simulink model "SITL"  (R2015a)
settings: Solver=ode3  StartTime=0.0  StopTime=tempofinal  FixedStep=0.02  RelTol=1e-3
values from neighbouring files (symbols this model uses):
  controle = 0    [main_quad.m]
  cq = 2.4086*10^(-7)    (= 2.4086e-07)    [main_quad.m]
  ct = 1.4341*10^(-5)    (= 1.4341e-05)    [main_quad.m]
  d = 0.26    [main_quad.m]
  g = 9.8065    [main_quad.m]
  J = [Jxx,Jyy,Jzz,Jm]    [main_quad.m]
  Ja = 5e-5    (= 5e-05)    [main_quad.m]
  k1 = 2.5    [main_quad.m]
  k2 = 6.2360    (= 6.236)    [main_quad.m]
  k3 = 6.2360    (= 6.236)    [main_quad.m]
  k4 = 0.4927    [main_quad.m]
  k5 = 1.6    [main_quad.m]
  k6 = 1.6    [main_quad.m]
  ke = kt    (= 0.024)    [main_quad.m]
  kt = 0.024    [main_quad.m]
  lambda1 = 1    [main_quad.m]
  lambda2 = 5    [main_quad.m]
  lambda3 = 5    [main_quad.m]
  lambda4 = 1/2    (= 0.5)    [main_quad.m]
  lambda5 = 1/4    (= 0.25)    [main_quad.m]
  lambda6 = 1/4    (= 0.25)    [main_quad.m]
  limit = [0.5 0.5 0.5 0.5]    [main_quad.m]
  limit_pos = [0.5 0.5]    [main_quad.m]
  m = 1.03    [main_quad.m]
  max_w = 733.03    [main_quad.m]
  Pitch_D = 0.019    [main_quad.m]
  Pitch_P = 0.019948    [main_quad.m]
  pos_D = -0.033991    [main_quad.m]
  pos_P = -0.005948    [main_quad.m]
  R = 0.2    [main_quad.m]    (also in plot_resultados.m = A(:,12))
  Roll_D = 0.019    [main_quad.m]
  Roll_P = 0.019948    [main_quad.m]
  w1_0 = w_hover    [main_quad.m]
  w2_0 = w_hover    [main_quad.m]
  w3_0 = w_hover    [main_quad.m]
  w4_0 = w_hover    [main_quad.m]
  X = A(:,1)    [plot_resultados.m]
  Yaw_D = 0.037200    (= 0.0372)    [main_quad.m]
  Yaw_P = 0.039055    [main_quad.m]
  Z_D = -0.682000    (= -0.682)    [main_quad.m]
  Z_P = -0.238672    [main_quad.m]
undefined symbols (not defined in the file or in its folder): selecting_parameters
libraries: dspnetwork x2, etargetslib x2
settings Model: Creator=Adriano  LastModifiedBy=Andre
settings DebuggingCC: UnderspecifiedInitializationDetection=Classic  MergeDetectMultiDrivingBlocksExec=none  SolverPrmCheckMsg=warning  StateNameClashWarn=warning
settings HardwareCC: ProdLargestAtomicInteger=Long  ProdLargestAtomicFloat=Double  ProdIntDivRoundTo=Floor  ProdEndianess=LittleEndian  ProdHWDeviceType=ARM Compatible->ARM Cortex
settings RTWCC: GenerateReport=on  LaunchReport=on
settings GRTTargetCC: CodeReplacementLibrary=GNU C99 extensions  RTWCAPISignals=on  RTWCAPIParams=on

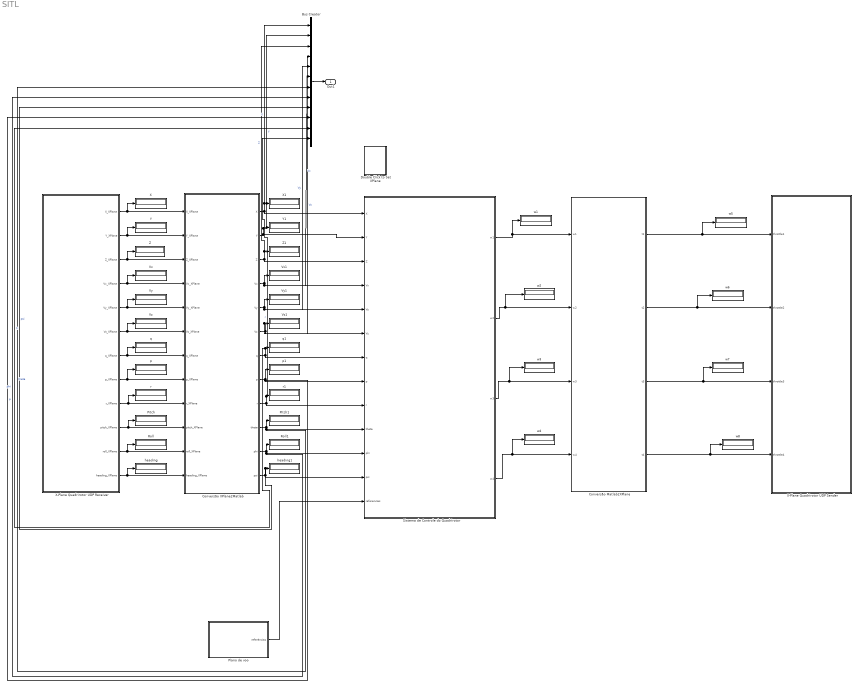
== system SITL ==
  Bus Creator : BusCreator  Inputs=12
  Conversão Matlab2XPlane : Subsystem
  Conversão XPlane2Matlab : Subsystem
  Double Click to Set XPlane : Subsystem  LoadFcn=selecting_parameters()
      settings: OpenFcn=selecting_parameters()
  Pitch : Display
  Pitch1 : Display
  Plano de voo : Subsystem
  Roll : Display
  Roll1 : Display
  Sistema de Controle do Quadrirotor : Subsystem
  Vx : Display
  Vx1 : Display
  Vy : Display
  Vy1 : Display
  Vz : Display
  Vz1 : Display
  X : Display
  X-Plane Quadrirotor UDP Receiver : Subsystem  AncestorBlock=X_Plane_Communication_Library/Fixed Wing/X-Plane Fixed Wing UDP Receiver  mask{ip_adress='127.0.0.1', port_number=49004}
      mask prompts: ip_adress "Local IP Adress (default: '127.0.0.1' )"; port_number "Output Port Number (defaut: '49004')"
      mask help: This block is configured to receiver data from a fixed wing aircraft on X-Plane Flight Simulator.
      mask Help: Contact adrianobittar@gmail.com
  X-Plane Quadrirotor UDP Sender : Subsystem  AncestorBlock=X_Plane_Communication_Library/Fixed Wing/X-Plane Fixed Wing UDP Sender  mask{ip_adress='127.0.0.1', port_number=49000}
      mask prompts: ip_adress "Local IP Adress (default: '127.0.0.1' )"; port_number "Output Port Number (defaut: '49000')"
      mask help: This block is configured to send data to a fixed wing aircraft on X-Plane Flight Simulator.
      mask Help: Contact adrianobittar@gmail.com
  X1 : Display
  Y : Display
  Y1 : Display
  Z : Display
  Z1 : Display
  heading : Display
  heading1 : Display
  p : Display
  p1 : Display
  q : Display
  q1 : Display
  r : Display
  r1 : Display
  w{1..8} (8 alike) : Display
  Out1 : Outport
  wires:
  X-Plane Quadrirotor UDP Receiver/10(pitch_XPlane) -> Pitch/1, Conversão XPlane2Matlab/10(pitch_XPlane)
  X-Plane Quadrirotor UDP Receiver/1("X_XPlane ") -> X/1, Conversão XPlane2Matlab/1(X_XPlane)
  X-Plane Quadrirotor UDP Receiver/2(Y_XPlane) -> Conversão XPlane2Matlab/2(Y_XPlane), Y/1
  X-Plane Quadrirotor UDP Receiver/3(Z_XPlane) -> Conversão XPlane2Matlab/3(Z_XPlane), Z/1
  X-Plane Quadrirotor UDP Receiver/4(Vx_XPlane) -> Conversão XPlane2Matlab/4(Vx_XPlane), Vx/1
  X-Plane Quadrirotor UDP Receiver/5(Vy_XPlane) -> Conversão XPlane2Matlab/5(Vy_XPlane), Vy/1
  X-Plane Quadrirotor UDP Receiver/8(p_XPlane) -> Conversão XPlane2Matlab/8(p_XPlane), p/1
  X-Plane Quadrirotor UDP Receiver/11(roll_XPlane) -> Conversão XPlane2Matlab/11(roll_XPlane), Roll/1
  X-Plane Quadrirotor UDP Receiver/9(r_XPlane) -> Conversão XPlane2Matlab/9(r_XPlane), r/1
  X-Plane Quadrirotor UDP Receiver/6(Vz_XPlane) -> Conversão XPlane2Matlab/6(Vz_XPlane), Vz/1
  X-Plane Quadrirotor UDP Receiver/12(heading_XPlane) -> Conversão XPlane2Matlab/12(heading_XPlane), heading/1
  X-Plane Quadrirotor UDP Receiver/7(q_XPlane) -> Conversão XPlane2Matlab/7(q_XPlane), q/1
  Sistema de Controle do Quadrirotor/3(w3) -> Conversão Matlab2XPlane/3(w3), w3/1
  Sistema de Controle do Quadrirotor/4(w4) -> Conversão Matlab2XPlane/4(w4), w4/1
  Sistema de Controle do Quadrirotor/2(w2) -> Conversão Matlab2XPlane/2(w2), w2/1
  Sistema de Controle do Quadrirotor/1(w1) -> Conversão Matlab2XPlane/1(w1), w1/1
  Conversão XPlane2Matlab/12(psi) -> Bus Creator/9, heading1/1, Sistema de Controle do Quadrirotor/12(psi)  "psi"
  Conversão XPlane2Matlab/11(phi) -> Bus Creator/8, Sistema de Controle do Quadrirotor/11(phi), Roll1/1  "phi"
  Conversão XPlane2Matlab/10(theta) -> Bus Creator/7, Sistema de Controle do Quadrirotor/10(theta), Pitch1/1  "theta"
  Conversão XPlane2Matlab/9(r) -> Bus Creator/12, r1/1, Sistema de Controle do Quadrirotor/9(r)  "r"
  Conversão XPlane2Matlab/8(p) -> Sistema de Controle do Quadrirotor/8(p), Bus Creator/10, p1/1  "p"
  Conversão XPlane2Matlab/7(q) -> Bus Creator/11, q1/1, Sistema de Controle do Quadrirotor/7(q)  "q"
  Conversão XPlane2Matlab/6(Vz) -> Bus Creator/6, Vz1/1, Sistema de Controle do Quadrirotor/6(Vz)  "Vz"
  Conversão XPlane2Matlab/5(Vy) -> Sistema de Controle do Quadrirotor/5(Vy), Bus Creator/5, Vy1/1  "Vy"
  Conversão XPlane2Matlab/4(Vx) -> Sistema de Controle do Quadrirotor/4(Vx), Bus Creator/4, Vx1/1  "Vx"
  Conversão XPlane2Matlab/3(Z) -> Bus Creator/3, Z1/1, Sistema de Controle do Quadrirotor/3(Z)  "Z"
  Conversão XPlane2Matlab/2(Y) -> Bus Creator/2, Y1/1, Sistema de Controle do Quadrirotor/2(Y)  "Y"
  Conversão XPlane2Matlab/1("X ") -> Bus Creator/1, X1/1, Sistema de Controle do Quadrirotor/1(X)  "X"
  Conversão Matlab2XPlane/1(t1) -> w5/1, X-Plane Quadrirotor UDP Sender/1(throttle1)
  Conversão Matlab2XPlane/2(t2) -> w6/1, X-Plane Quadrirotor UDP Sender/2(throttle2)
  Conversão Matlab2XPlane/3(t3) -> w7/1, X-Plane Quadrirotor UDP Sender/3(throttle3)
  Conversão Matlab2XPlane/4(t4) -> w8/1, X-Plane Quadrirotor UDP Sender/4(throttle4)
  Plano de voo/1("referências ") -> Sistema de Controle do Quadrirotor/13(referencias)
  Bus Creator/1 -> Out1/1

== system SITL/Conversão Matlab2XPlane ==
  w1 : Inport
  w2 : Inport  Port=2
  w3 : Inport  Port=3
  w4 : Inport  Port=4
  MATLAB Function : MATLAB Function  TreatAsAtomicUnit=on
  t1 : Outport
  t2 : Outport  Port=2
  t3 : Outport  Port=3
  t4 : Outport  Port=4
  wires:
  w1/1 -> MATLAB Function/1(w1)
  w2/1 -> MATLAB Function/2(w2)
  w3/1 -> MATLAB Function/3(w3)
  w4/1 -> MATLAB Function/4(w4)
  MATLAB Function/1(t1) -> t1/1
  MATLAB Function/2(t2) -> t2/1
  MATLAB Function/3(t3) -> t3/1
  MATLAB Function/4(t4) -> t4/1

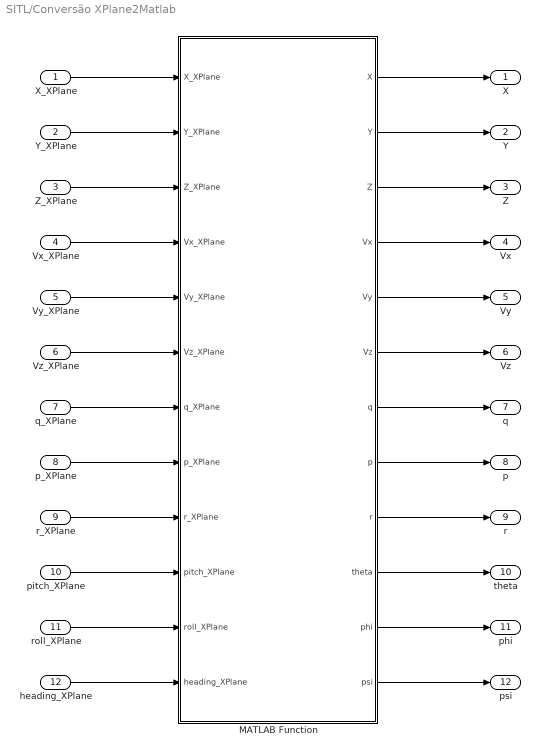
== system SITL/Conversão XPlane2Matlab ==
  X_XPlane : Inport
  Y_XPlane : Inport  Port=2
  Z_XPlane : Inport  Port=3
  Vx_XPlane : Inport  Port=4
  Vy_XPlane : Inport  Port=5
  Vz_XPlane : Inport  Port=6
  q_XPlane : Inport  Port=7
  p_XPlane : Inport  Port=8
  r_XPlane : Inport  Port=9
  pitch_XPlane : Inport  Port=10
  roll_XPlane : Inport  Port=11
  heading_XPlane : Inport  Port=12
  MATLAB Function : MATLAB Function  TreatAsAtomicUnit=on
  "X " : Outport
  Y : Outport  Port=2
  Z : Outport  Port=3
  Vx : Outport  Port=4
  Vy : Outport  Port=5
  Vz : Outport  Port=6
  q : Outport  Port=7
  p : Outport  Port=8
  r : Outport  Port=9
  theta : Outport  Port=10
  phi : Outport  Port=11
  psi : Outport  Port=12
  wires:
  MATLAB Function/12(psi) -> psi/1
  MATLAB Function/11(phi) -> phi/1
  MATLAB Function/10(theta) -> theta/1
  MATLAB Function/9(r) -> r/1
  MATLAB Function/8(p) -> p/1
  MATLAB Function/7(q) -> q/1
  MATLAB Function/6(Vz) -> Vz/1
  MATLAB Function/5(Vy) -> Vy/1
  MATLAB Function/4(Vx) -> Vx/1
  MATLAB Function/3(Z) -> Z/1
  MATLAB Function/2(Y) -> Y/1
  MATLAB Function/1(X) -> "X "/1
  X_XPlane/1 -> MATLAB Function/1(X_XPlane)
  Y_XPlane/1 -> MATLAB Function/2(Y_XPlane)
  Z_XPlane/1 -> MATLAB Function/3(Z_XPlane)
  Vx_XPlane/1 -> MATLAB Function/4(Vx_XPlane)
  Vy_XPlane/1 -> MATLAB Function/5(Vy_XPlane)
  Vz_XPlane/1 -> MATLAB Function/6(Vz_XPlane)
  q_XPlane/1 -> MATLAB Function/7(q_XPlane)
  p_XPlane/1 -> MATLAB Function/8(p_XPlane)
  r_XPlane/1 -> MATLAB Function/9(r_XPlane)
  pitch_XPlane/1 -> MATLAB Function/10(pitch_XPlane)
  roll_XPlane/1 -> MATLAB Function/11(roll_XPlane)
  heading_XPlane/1 -> MATLAB Function/12(heading_XPlane)

== system SITL/Double Click to Set XPlane ==

== system SITL/Plano de voo ==
  Gain1 : Gain
  Gain2 : Gain
  Gain3 : Gain  Gain=-1
  Gain4 : Gain
  Mux : Mux
  Step1 : Step  Time=30  After=150*pi/180  SampleTime=0
  Step2 : Step  Time=0  After=6  SampleTime=0
  Step_x : Step  Time=20  After=15  SampleTime=0
  Step_y : Step  Time=10  After=15  SampleTime=0
  "referências " : Outport
  wires:
  Mux/1 -> "referências "/1
  Gain3/1 -> Mux/3  "ref_z"
  Gain2/1 -> Mux/2  "ref_y"
  Gain4/1 -> Mux/1  "ref_x"
  Gain1/1 -> Mux/4  "ref_psi"
  Step1/1 -> Gain1/1
  Step2/1 -> Gain3/1
  Step_y/1 -> Gain2/1
  Step_x/1 -> Gain4/1

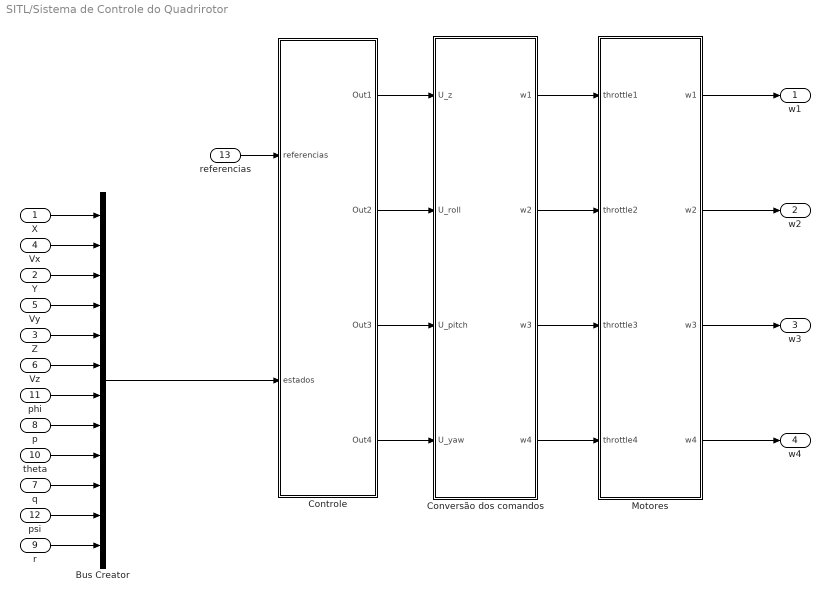
== system SITL/Sistema de Controle do Quadrirotor ==
  X : Inport
  Y : Inport  Port=2
  Z : Inport  Port=3
  Vx : Inport  Port=4
  Vy : Inport  Port=5
  Vz : Inport  Port=6
  q : Inport  Port=7
  p : Inport  Port=8
  r : Inport  Port=9
  theta : Inport  Port=10
  phi : Inport  Port=11
  psi : Inport  Port=12
  referencias : Inport  Port=13
  Bus Creator : BusCreator  Inputs=12
  Controle : Subsystem
  Conversão dos comandos : Subsystem
  Motores : Subsystem
  w1 : Outport
  w2 : Outport  Port=2
  w3 : Outport  Port=3
  w4 : Outport  Port=4
  wires:
  Conversão dos comandos/1(w1) -> Motores/1(throttle1)
  Conversão dos comandos/2(w2) -> Motores/2(throttle2)
  Conversão dos comandos/3(w3) -> Motores/3(throttle3)
  Conversão dos comandos/4(w4) -> Motores/4(throttle4)
  Controle/1(Out1) -> Conversão dos comandos/1(U_z)
  Controle/2(Out2) -> Conversão dos comandos/2(U_roll)
  Controle/3(Out3) -> Conversão dos comandos/3(U_pitch)
  Controle/4(Out4) -> Conversão dos comandos/4(U_yaw)
  referencias/1 -> Controle/1(referencias)
  X/1 -> Bus Creator/1
  Bus Creator/1 -> Controle/2(estados)
  Vx/1 -> Bus Creator/2
  Y/1 -> Bus Creator/3
  Vy/1 -> Bus Creator/4
  Z/1 -> Bus Creator/5
  Vz/1 -> Bus Creator/6
  phi/1 -> Bus Creator/7
  p/1 -> Bus Creator/8
  theta/1 -> Bus Creator/9
  q/1 -> Bus Creator/10
  psi/1 -> Bus Creator/11
  r/1 -> Bus Creator/12
  Motores/1(w1) -> w1/1
  Motores/2(w2) -> w2/1
  Motores/3(w3) -> w3/1
  Motores/4(w4) -> w4/1

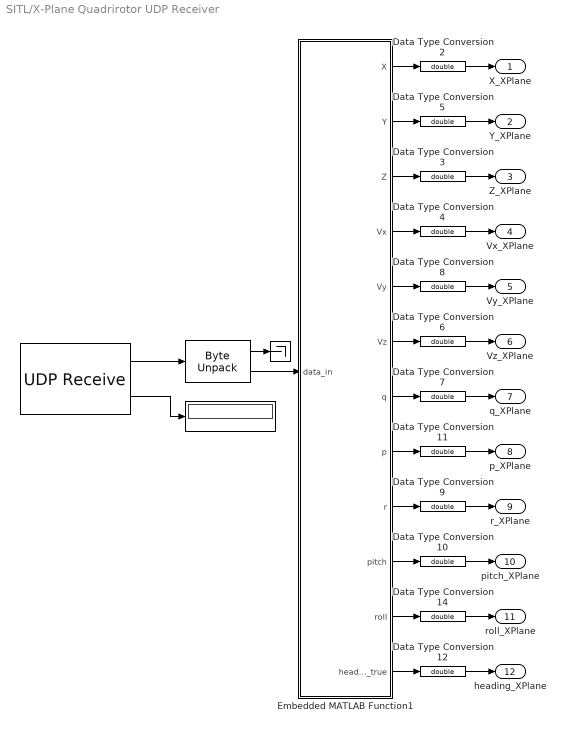
== system SITL/X-Plane Quadrirotor UDP Receiver ==
  " " : Display
  " " : Terminator
  "    " : dspnetwork/UDP Receive  localURL='0.0.0.0'  localPort=port_number  remoteURL=ip_adress  remotePort=-1  recvBufferSize=8192  dims=113  signalDatatype=uint8  isVarSize=off  showBlockingTime=on  blockingTime=1  sampletime=0.02  blockPlatform=WINDOWS
  "     " : etargetslib/Byte Unpack  dimensions={5,[9,3]}  datatypes={'uint8','single'}  byteAlign=1
  Data Type Conversion{2..12,14} (12 alike) : DataTypeConversion  OutDataTypeStr=double  SaturateOnIntegerOverflow=on
  Embedded MATLAB Function1 : MATLAB Function  TreatAsAtomicUnit=on
  "X_XPlane " : Outport
  Y_XPlane : Outport  Port=2
  Z_XPlane : Outport  Port=3
  Vx_XPlane : Outport  Port=4
  Vy_XPlane : Outport  Port=5
  Vz_XPlane : Outport  Port=6
  q_XPlane : Outport  Port=7
  p_XPlane : Outport  Port=8
  r_XPlane : Outport  Port=9
  pitch_XPlane : Outport  Port=10
  roll_XPlane : Outport  Port=11
  heading_XPlane : Outport  Port=12
  wires:
  Data Type Conversion11/1 -> p_XPlane/1
  Data Type Conversion14/1 -> roll_XPlane/1
  Data Type Conversion12/1 -> heading_XPlane/1
  Data Type Conversion7/1 -> q_XPlane/1
  Data Type Conversion6/1 -> Vz_XPlane/1
  Data Type Conversion4/1 -> Vx_XPlane/1
  Data Type Conversion3/1 -> Z_XPlane/1
  Data Type Conversion8/1 -> Vy_XPlane/1
  Data Type Conversion5/1 -> Y_XPlane/1
  Data Type Conversion2/1 -> "X_XPlane "/1
  Embedded MATLAB Function1/1(X) -> Data Type Conversion2/1
  Embedded MATLAB Function1/2(Y) -> Data Type Conversion5/1
  Embedded MATLAB Function1/3(Z) -> Data Type Conversion3/1
  Embedded MATLAB Function1/4(Vx) -> Data Type Conversion4/1
  Embedded MATLAB Function1/5(Vy) -> Data Type Conversion8/1
  Embedded MATLAB Function1/6(Vz) -> Data Type Conversion6/1
  Embedded MATLAB Function1/7(q) -> Data Type Conversion7/1
  Embedded MATLAB Function1/8(p) -> Data Type Conversion11/1
  Embedded MATLAB Function1/9(r) -> Data Type Conversion9/1
  Embedded MATLAB Function1/10(pitch) -> Data Type Conversion10/1
  Embedded MATLAB Function1/11(roll) -> Data Type Conversion14/1
  Embedded MATLAB Function1/12(heading_true) -> Data Type Conversion12/1
  "     "/1 -> " "/1
  "    "/2 -> " "/1
  Data Type Conversion10/1 -> pitch_XPlane/1
  "    "/1 -> "     "/1
  Data Type Conversion9/1 -> r_XPlane/1
  "     "/2 -> Embedded MATLAB Function1/1(data_in)

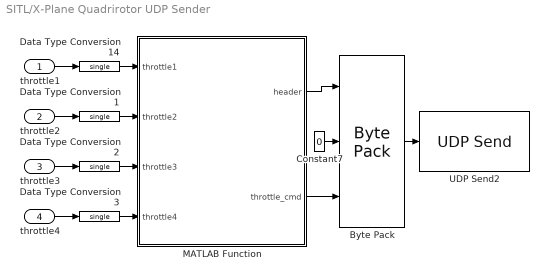
== system SITL/X-Plane Quadrirotor UDP Sender ==
  throttle1 : Inport
  throttle2 : Inport  Port=2
  throttle3 : Inport  Port=3
  throttle4 : Inport  Port=4
  Byte Pack : etargetslib/Byte Pack  datatypes={'single','uint8','single'}  byteAlign=1
  Constant7 : Constant  Value=0  OutDataTypeStr=uint8
  Data Type Conversion{1..3,14} (4 alike) : DataTypeConversion  OutDataTypeStr=single  SaturateOnIntegerOverflow=on
  MATLAB Function : MATLAB Function  TreatAsAtomicUnit=on
  UDP Send2 : dspnetwork/UDP Send  remoteURL=ip_adress  remotePort=port_number  localURL='255.255.255.255'  localPortSource=Automatically determine  localPort=-1  sampletime=-1  blockPlatform=HOST  separateLengthPort=0
  wires:
  Byte Pack/1 -> UDP Send2/1
  MATLAB Function/1(header) -> Byte Pack/1
  Data Type Conversion14/1 -> MATLAB Function/1(throttle1)
  throttle1/1 -> Data Type Conversion14/1
  Constant7/1 -> Byte Pack/2
  Data Type Conversion1/1 -> MATLAB Function/2(throttle2)
  Data Type Conversion2/1 -> MATLAB Function/3(throttle3)
  Data Type Conversion3/1 -> MATLAB Function/4(throttle4)
  throttle2/1 -> Data Type Conversion1/1
  throttle3/1 -> Data Type Conversion2/1
  throttle4/1 -> Data Type Conversion3/1
  MATLAB Function/2(throttle_cmd) -> Byte Pack/3

== system SITL/Sistema de Controle do Quadrirotor/Controle ==
  note: 0: controle Sliding Mode
      | 1: controle PD
  referencias : Inport
  estados : Inport  Port=2
  Constant : Constant  Value=0
  Controlador PD : Subsystem
  Controlador sliding mode : Subsystem
  Demux : Demux
  Switch : Switch  Criteria=u2 > Threshold
  Out1 : Outport
  Out2 : Outport  Port=2
  Out3 : Outport  Port=3
  Out4 : Outport  Port=4
  wires:
  referencias/1 -> Controlador sliding mode/1(Referências), Controlador PD/1(Referências)
  estados/1 -> Controlador sliding mode/2(Estados), Controlador PD/2(Estados)
  Switch/1 -> Demux/1
  Demux/1 -> Out1/1  "U_T"
  Demux/2 -> Out2/1  "U_L"
  Constant/1 -> Switch/2
  Demux/3 -> Out3/1  "U_M"
  Demux/4 -> Out4/1  "U_N"
  Controlador PD/1(Out1) -> Switch/1
  Controlador sliding mode/1(Out1) -> Switch/3

== system SITL/Sistema de Controle do Quadrirotor/Conversão dos comandos ==
  U_z : Inport
  U_roll : Inport  Port=2
  U_pitch : Inport  Port=3
  U_yaw : Inport  Port=4
  Constant1 : Constant  Value=ct
  Constant2 : Constant  Value=cq
  Constant4 : Constant  Value=d
  MATLAB Function : MATLAB Function  TreatAsAtomicUnit=on
  w1 : Outport
  w2 : Outport  Port=2
  w3 : Outport  Port=3
  w4 : Outport  Port=4
  wires:
  U_pitch/1 -> MATLAB Function/3(u_M)
  U_z/1 -> MATLAB Function/1(u_T)
  U_yaw/1 -> MATLAB Function/4(u_N)
  Constant4/1 -> MATLAB Function/5(d)
  Constant1/1 -> MATLAB Function/6(ct)
  Constant2/1 -> MATLAB Function/7(cq)
  U_roll/1 -> MATLAB Function/2(u_L)
  MATLAB Function/1(w1d) -> w1/1  "w1d"
  MATLAB Function/2(w2d) -> w2/1  "w2d"
  MATLAB Function/3(w3d) -> w3/1  "w3d"
  MATLAB Function/4(w4d) -> w4/1  "w4d"

== system SITL/Sistema de Controle do Quadrirotor/Motores ==
  throttle1 : Inport
  throttle2 : Inport  Port=2
  throttle3 : Inport  Port=3
  throttle4 : Inport  Port=4
  Motor 1 : Subsystem
  Motor 2 : Subsystem
  Motor 3 : Subsystem
  Motor 4 : Subsystem
  w1 : Outport
  w2 : Outport  Port=2
  w3 : Outport  Port=3
  w4 : Outport  Port=4
  wires:
  throttle1/1 -> Motor 1/1(In1)  "w1d"
  throttle3/1 -> Motor 3/1(In1)  "w3d"
  throttle4/1 -> Motor 4/1(In1)  "w4d"
  throttle2/1 -> Motor 2/1(In1)  "w2d"
  Motor 1/1(Out1) -> w1/1  "w1"
  Motor 3/1(Out1) -> w3/1  "w3"
  Motor 4/1(Out1) -> w4/1  "w4"
  Motor 2/1(Out1) -> w2/1  "w2"

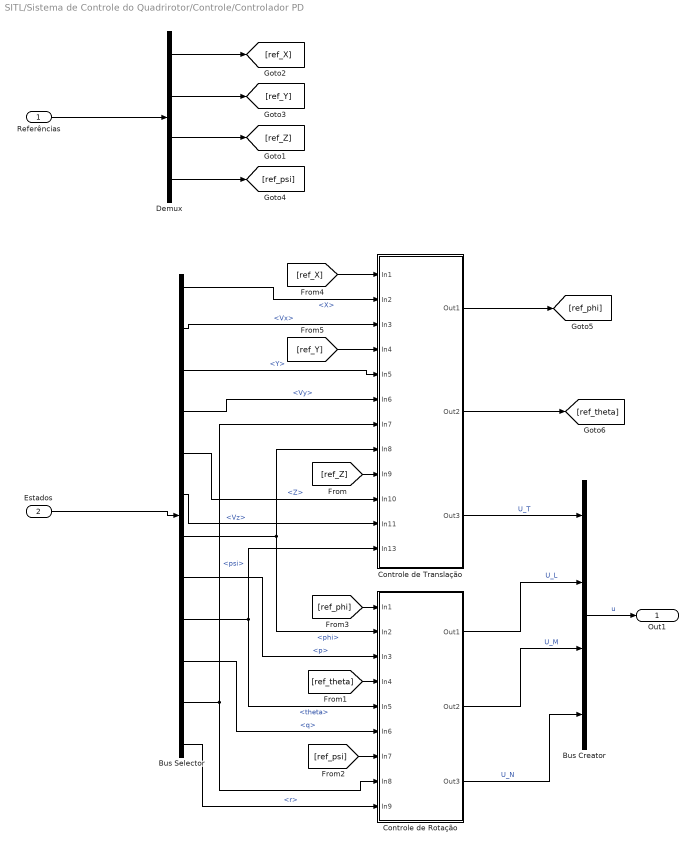
== system SITL/Sistema de Controle do Quadrirotor/Controle/Controlador PD ==
  Referências : Inport
  Estados : Inport  Port=2
  Bus Creator : BusCreator
  Bus Selector : BusSelector  OutputSignals=X,Vx,Y,Vy,Z,Vz,phi,p,theta,q,psi,r
  Controle de Rotação : Subsystem
  Controle de Translação : Subsystem
  Demux : Demux
  Out1 : Outport
  wires:
  Demux/4 -> [ref_psi]
  Bus Creator/1 -> Out1/1  "u"
  Demux/1 -> [ref_X]
  Demux/2 -> [ref_Y]
  Demux/3 -> [ref_Z]
  [ref_phi] -> Controle de Rotação/1(In1)
  [ref_theta] -> Controle de Rotação/4(In4)
  Controle de Rotação/1(Out1) -> Bus Creator/2  "U_L"
  Controle de Rotação/2(Out2) -> Bus Creator/3  "U_M"
  Controle de Rotação/3(Out3) -> Bus Creator/4  "U_N"
  [ref_X] -> Controle de Translação/1(In1)
  Controle de Translação/3(Out3) -> Bus Creator/1  "U_T"
  [ref_Y] -> Controle de Translação/4(In4)
  [ref_Z] -> Controle de Translação/9(In9)
  Bus Selector/1 -> Controle de Translação/2(In2)  "<X>"
  Bus Selector/2 -> Controle de Translação/3(In3)  "<Vx>"
  Bus Selector/3 -> Controle de Translação/5(In5)  "<Y>"
  Bus Selector/4 -> Controle de Translação/6(In6)  "<Vy>"
  Bus Selector/5 -> Controle de Translação/10(In10)  "<Z>"
  Bus Selector/6 -> Controle de Translação/11(In11)  "<Vz>"
  [ref_psi] -> Controle de Rotação/7(In7)
  Referências/1 -> Demux/1
  Estados/1 -> Bus Selector/1
  Controle de Translação/1(Out1) -> [ref_phi]
  Controle de Translação/2(Out2) -> [ref_theta]
  Bus Selector/12 -> Controle de Rotação/9(In9)  "<r>"
  Bus Selector/10 -> Controle de Rotação/6(In6)  "<q>"
  Bus Selector/9 -> Controle de Rotação/5(In5), Controle de Translação/12(In13)  "<theta>"
  Bus Selector/8 -> Controle de Rotação/3(In3)  "<p>"
  Bus Selector/7 -> Controle de Translação/8(In8), Controle de Rotação/2(In2)  "<phi>"
  Bus Selector/11 -> Controle de Rotação/8(In8), Controle de Translação/7(In7)  "<psi>"

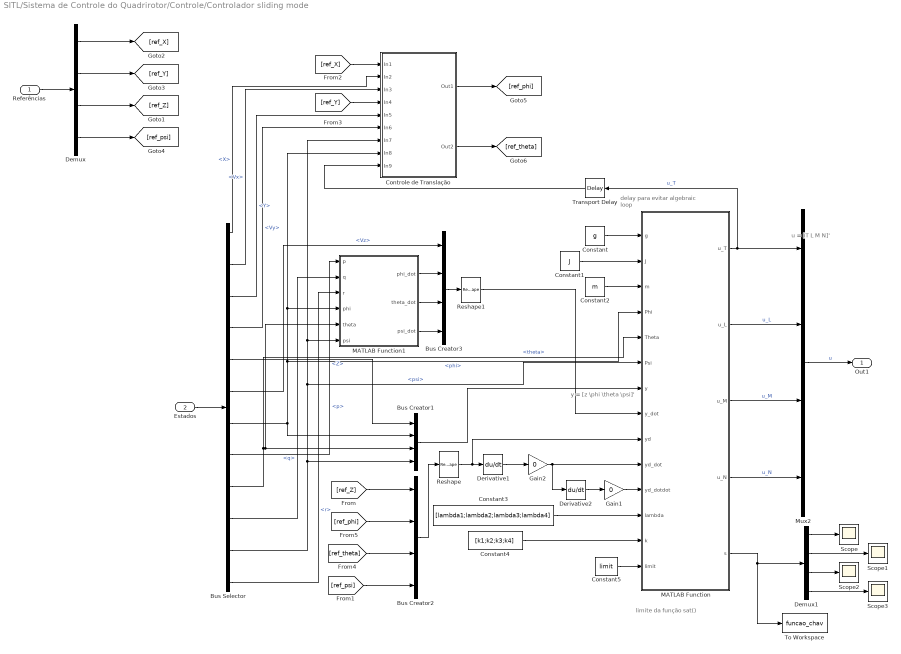
== system SITL/Sistema de Controle do Quadrirotor/Controle/Controlador sliding mode ==
  note: limite da função sat()
  note: delay para evitar
      |  algebraic loop
  note: y = [z \phi \theta \psi]'
  note: u = [T L M N]'
  Referências : Inport
  Estados : Inport  Port=2
  Bus Creator1 : BusCreator
  Bus Creator2 : BusCreator
  Bus Creator3 : BusCreator
  Bus Selector : BusSelector  OutputSignals=X,Vx,Y,Vy,Z,Vz,phi,p,theta,q,psi,r
  Constant : Constant  Value=g
  Constant1 : Constant  Value=J
  Constant2 : Constant  Value=m
  Constant3 : Constant  Value=[lambda1;lambda2;lambda3;lambda4]
  Constant4 : Constant  Value=[k1;k2;k3;k4]
  Constant5 : Constant  Value=limit
  Controle de Translação : Subsystem
  Demux : Demux
  Demux1 : Demux
  Derivative1 : Derivative
  Derivative2 : Derivative
  Gain1 : Gain  Gain=0
  Gain2 : Gain  Gain=0
  MATLAB Function : MATLAB Function  TreatAsAtomicUnit=on
  MATLAB Function1 : MATLAB Function  TreatAsAtomicUnit=on
  Mux2 : Mux
  Reshape : Reshape  OutputDimensionality=Customize  OutputDimensions=[4,1]
  Reshape1 : Reshape  OutputDimensionality=Customize  OutputDimensions=[4,1]
  Scope{,1..3} (4 alike) : Scope
      Scope settings: TimeRange=100  YMin=-1
      Scope1 settings: TimeRange=100  YMin=-1  SaveName=ScopeData4
      Scope2 settings: TimeRange=100  YMin=-1  SaveName=ScopeData5
      Scope3 settings: TimeRange=100  YMin=-1  SaveName=ScopeData6
  To Workspace : ToWorkspace  VariableName=funcao_chav  SampleTime=-1
  Transport Delay : TransportDelay  DelayTime=0.01  InitialOutput=m*g
  Out1 : Outport
  wires:
  Demux/4 -> [ref_psi]
  Estados/1 -> Bus Selector/1
  Referências/1 -> Demux/1
  Demux/1 -> [ref_X]
  Demux/2 -> [ref_Y]
  Demux/3 -> [ref_Z]
  Constant/1 -> MATLAB Function/1(g)
  Constant1/1 -> MATLAB Function/2(J)
  Constant2/1 -> MATLAB Function/3(m)
  Bus Selector/5 -> Bus Creator1/1  "<Z>"
  Bus Selector/11 -> Bus Creator1/4, Controle de Translação/7(In7), MATLAB Function1/6(psi), MATLAB Function/6(Psi)  "<psi>"
  Constant3/1 -> MATLAB Function/12(lambda)
  Constant4/1 -> MATLAB Function/13(k)
  Derivative2/1 -> Gain1/1
  Mux2/1 -> Out1/1  "u"
  MATLAB Function/1(u_T) -> Mux2/1, Transport Delay/1  "u_T"
  MATLAB Function/2(u_L) -> Mux2/2  "u_L"
  MATLAB Function/4(u_N) -> Mux2/4  "u_N"
  MATLAB Function/3(u_M) -> Mux2/3  "u_M"
  Gain1/1 -> MATLAB Function/11(yd_dotdot)
  Gain2/1 -> Derivative2/1, MATLAB Function/10(yd_dot)
  Bus Selector/2 -> Controle de Translação/3(In3)  "<Vx>"
  Bus Selector/3 -> Controle de Translação/5(In5)  "<Y>"
  Bus Selector/4 -> Controle de Translação/6(In6)  "<Vy>"
  [ref_X] -> Controle de Translação/1(In1)
  [ref_Y] -> Controle de Translação/4(In4)
  [ref_Z] -> Bus Creator2/1
  [ref_psi] -> Bus Creator2/4
  Bus Creator2/1 -> Reshape/1
  [ref_theta] -> Bus Creator2/3
  [ref_phi] -> Bus Creator2/2
  Bus Creator1/1 -> MATLAB Function/7(y)
  Controle de Translação/1(Out1) -> [ref_phi]
  Controle de Translação/2(Out2) -> [ref_theta]
  Reshape/1 -> MATLAB Function/9(yd), Derivative1/1
  Transport Delay/1 -> Controle de Translação/9(In9)
  Constant5/1 -> MATLAB Function/14(limit)
  Bus Selector/6 -> Bus Creator3/1  "<Vz>"
  MATLAB Function1/1(phi_dot) -> Bus Creator3/2
  MATLAB Function1/2(theta_dot) -> Bus Creator3/3
  MATLAB Function1/3(psi_dot) -> Bus Creator3/4
  Bus Creator3/1 -> Reshape1/1
  Reshape1/1 -> MATLAB Function/8(y_dot)
  MATLAB Function/5(s) -> Demux1/1, To Workspace/1
  Derivative1/1 -> Gain2/1
  Demux1/1 -> Scope/1
  Demux1/2 -> Scope1/1
  Demux1/3 -> Scope2/1
  Demux1/4 -> Scope3/1
  Bus Selector/1 -> Controle de Translação/2(In2)  "<X>"
  Bus Selector/7 -> MATLAB Function/4(Phi), MATLAB Function1/4(phi), Controle de Translação/8(In8), Bus Creator1/2  "<phi>"
  Bus Selector/12 -> MATLAB Function1/3(r)  "<r>"
  Bus Selector/10 -> MATLAB Function1/2(q)  "<q>"
  Bus Selector/8 -> MATLAB Function1/1(p)  "<p>"
  Bus Selector/9 -> MATLAB Function/5(Theta), MATLAB Function1/5(theta), Bus Creator1/3  "<theta>"

== system SITL/Sistema de Controle do Quadrirotor/Motores/Motor 1 ==
  In1 : Inport
  Constant : Constant  Value=ke
  Constant1 : Constant  Value=cq
  Constant2 : Constant  Value=kt
  Constant3 : Constant  Value=R
  Constant4 : Constant  Value=Ja
  Integrator : Integrator  InitialCondition=w1_0
  MATLAB Function : MATLAB Function  TreatAsAtomicUnit=on
  Saturation : Saturate  UpperLimit=max_w  LowerLimit=0
  Out1 : Outport
  wires:
  MATLAB Function/1(wder) -> Integrator/1
  Saturation/1 -> MATLAB Function/2(w), Out1/1  "w1"
  Integrator/1 -> Saturation/1
  Constant/1 -> MATLAB Function/3(ke)
  Constant1/1 -> MATLAB Function/4(cq)
  Constant2/1 -> MATLAB Function/5(kt)
  Constant3/1 -> MATLAB Function/6(R)
  Constant4/1 -> MATLAB Function/7(Ja)
  In1/1 -> MATLAB Function/1(wd)

== system SITL/Sistema de Controle do Quadrirotor/Motores/Motor 2 ==
  In1 : Inport
  Constant : Constant  Value=ke
  Constant1 : Constant  Value=cq
  Constant2 : Constant  Value=kt
  Constant3 : Constant  Value=R
  Constant4 : Constant  Value=Ja
  Integrator : Integrator  InitialCondition=w2_0
  MATLAB Function : MATLAB Function  TreatAsAtomicUnit=on
  Saturation : Saturate  UpperLimit=max_w  LowerLimit=0
  Out1 : Outport
  wires:
  MATLAB Function/1(wder) -> Integrator/1
  Saturation/1 -> MATLAB Function/2(w), Out1/1  "w2"
  Integrator/1 -> Saturation/1
  Constant/1 -> MATLAB Function/3(ke)
  Constant1/1 -> MATLAB Function/4(cq)
  Constant2/1 -> MATLAB Function/5(kt)
  Constant3/1 -> MATLAB Function/6(R)
  Constant4/1 -> MATLAB Function/7(Ja)
  In1/1 -> MATLAB Function/1(wd)

== system SITL/Sistema de Controle do Quadrirotor/Motores/Motor 3 ==
  In1 : Inport
  Constant : Constant  Value=ke
  Constant1 : Constant  Value=cq
  Constant2 : Constant  Value=kt
  Constant3 : Constant  Value=R
  Constant4 : Constant  Value=Ja
  Integrator : Integrator  InitialCondition=w3_0
  MATLAB Function : MATLAB Function  TreatAsAtomicUnit=on
  Saturation : Saturate  UpperLimit=max_w  LowerLimit=0
  Out1 : Outport
  wires:
  MATLAB Function/1(wder) -> Integrator/1
  Saturation/1 -> MATLAB Function/2(w), Out1/1  "w3"
  Integrator/1 -> Saturation/1
  Constant/1 -> MATLAB Function/3(ke)
  Constant1/1 -> MATLAB Function/4(cq)
  Constant2/1 -> MATLAB Function/5(kt)
  Constant3/1 -> MATLAB Function/6(R)
  Constant4/1 -> MATLAB Function/7(Ja)
  In1/1 -> MATLAB Function/1(wd)

== system SITL/Sistema de Controle do Quadrirotor/Motores/Motor 4 ==
  In1 : Inport
  Constant : Constant  Value=ke
  Constant1 : Constant  Value=cq
  Constant2 : Constant  Value=kt
  Constant3 : Constant  Value=R
  Constant4 : Constant  Value=Ja
  Integrator : Integrator  InitialCondition=w4_0
  MATLAB Function : MATLAB Function  TreatAsAtomicUnit=on
  Saturation : Saturate  UpperLimit=max_w  LowerLimit=0
  Out1 : Outport
  wires:
  MATLAB Function/1(wder) -> Integrator/1
  Saturation/1 -> MATLAB Function/2(w), Out1/1  "w4"
  Integrator/1 -> Saturation/1
  Constant/1 -> MATLAB Function/3(ke)
  Constant1/1 -> MATLAB Function/4(cq)
  Constant2/1 -> MATLAB Function/5(kt)
  Constant3/1 -> MATLAB Function/6(R)
  Constant4/1 -> MATLAB Function/7(Ja)
  In1/1 -> MATLAB Function/1(wd)

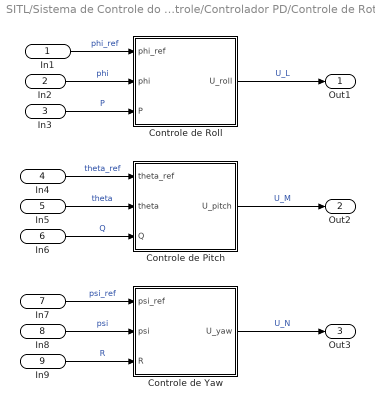
== system SITL/Sistema de Controle do Quadrirotor/Controle/Controlador PD/Controle de Rotação ==
  In1 : Inport
  In2 : Inport  Port=2
  In3 : Inport  Port=3
  In4 : Inport  Port=4
  In5 : Inport  Port=5
  In6 : Inport  Port=6
  In7 : Inport  Port=7
  In8 : Inport  Port=8
  In9 : Inport  Port=9
  Controle de Pitch : Subsystem
  Controle de Roll : Subsystem
  Controle de Yaw : Subsystem
  Out1 : Outport
  Out2 : Outport  Port=2
  Out3 : Outport  Port=3
  wires:
  In2/1 -> Controle de Roll/2(phi)  "phi"
  In4/1 -> Controle de Pitch/1(theta_ref)  "theta_ref"
  In3/1 -> Controle de Roll/3(P)  "P"
  In1/1 -> Controle de Roll/1(phi_ref)  "phi_ref"
  Controle de Roll/1(U_roll) -> Out1/1  "U_L"
  Controle de Pitch/1(U_pitch) -> Out2/1  "U_M"
  Controle de Yaw/1(U_yaw) -> Out3/1  "U_N"
  In5/1 -> Controle de Pitch/2(theta)  "theta"
  In6/1 -> Controle de Pitch/3(Q)  "Q"
  In7/1 -> Controle de Yaw/1(psi_ref)  "psi_ref"
  In8/1 -> Controle de Yaw/2(psi)  "psi"
  In9/1 -> Controle de Yaw/3(R)  "R"

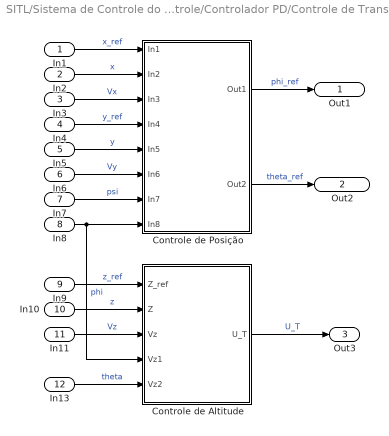
== system SITL/Sistema de Controle do Quadrirotor/Controle/Controlador PD/Controle de Translação ==
  In1 : Inport
  In2 : Inport  Port=2
  In3 : Inport  Port=3
  In4 : Inport  Port=4
  In5 : Inport  Port=5
  In6 : Inport  Port=6
  In7 : Inport  Port=7
  In8 : Inport  Port=8
  In9 : Inport  Port=9
  In10 : Inport  Port=10
  In11 : Inport  Port=11
  In13 : Inport  Port=12
  Controle de Altitude : Subsystem
  Controle de Posição : Subsystem
  Out1 : Outport
  Out2 : Outport  Port=2
  Out3 : Outport  Port=3
  wires:
  Controle de Altitude/1(U_T) -> Out3/1  "U_T"
  Controle de Posição/1(Out1) -> Out1/1  "phi_ref"
  Controle de Posição/2(Out2) -> Out2/1  "theta_ref"
  In1/1 -> Controle de Posição/1(In1)  "x_ref"
  In2/1 -> Controle de Posição/2(In2)  "x"
  In3/1 -> Controle de Posição/3(In3)  "Vx"
  In4/1 -> Controle de Posição/4(In4)  "y_ref"
  In5/1 -> Controle de Posição/5(In5)  "y"
  In6/1 -> Controle de Posição/6(In6)  "Vy"
  In7/1 -> Controle de Posição/7(In7)  "psi"
  In9/1 -> Controle de Altitude/1(Z_ref)  "z_ref"
  In10/1 -> Controle de Altitude/2(Z)  "z"
  In11/1 -> Controle de Altitude/3(Vz)  "Vz"
  In8/1 -> Controle de Altitude/4(Vz1), Controle de Posição/8(In8)  "phi"
  In13/1 -> Controle de Altitude/5(Vz2)  "theta"

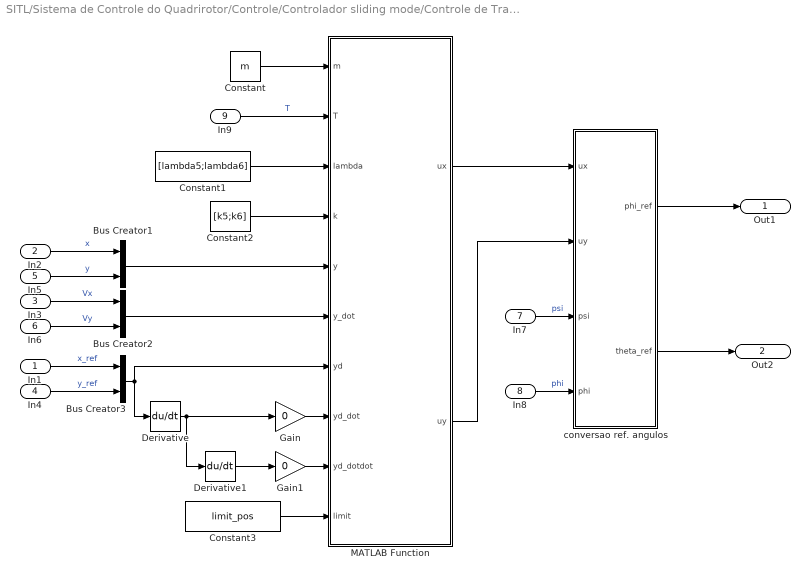
== system SITL/Sistema de Controle do Quadrirotor/Controle/Controlador sliding mode/Controle de Translação ==
  In1 : Inport
  In2 : Inport  Port=2
  In3 : Inport  Port=3
  In4 : Inport  Port=4
  In5 : Inport  Port=5
  In6 : Inport  Port=6
  In7 : Inport  Port=7
  In8 : Inport  Port=8
  In9 : Inport  Port=9
  Bus Creator1 : BusCreator  Inputs=2
  Bus Creator2 : BusCreator  Inputs=2
  Bus Creator3 : BusCreator  Inputs=2
  Constant : Constant  Value=m
  Constant1 : Constant  Value=[lambda5;lambda6]
  Constant2 : Constant  Value=[k5;k6]
  Constant3 : Constant  Value=limit_pos
  Derivative : Derivative
  Derivative1 : Derivative
  Gain : Gain  Gain=0
  Gain1 : Gain  Gain=0
  MATLAB Function : MATLAB Function  TreatAsAtomicUnit=on
  conversao ref. angulos : MATLAB Function  TreatAsAtomicUnit=on
  Out1 : Outport
  Out2 : Outport  Port=2
  wires:
  MATLAB Function/1(ux) -> conversao ref. angulos/1(ux)
  conversao ref. angulos/1(phi_ref) -> Out1/1
  conversao ref. angulos/2(theta_ref) -> Out2/1
  Constant/1 -> MATLAB Function/1(m)
  Constant1/1 -> MATLAB Function/3(lambda)
  Constant2/1 -> MATLAB Function/4(k)
  Bus Creator1/1 -> MATLAB Function/5(y)
  In2/1 -> Bus Creator1/1  "x"
  In5/1 -> Bus Creator1/2  "y"
  Bus Creator2/1 -> MATLAB Function/6(y_dot)
  In3/1 -> Bus Creator2/1  "Vx"
  In6/1 -> Bus Creator2/2  "Vy"
  Bus Creator3/1 -> MATLAB Function/7(yd), Derivative/1
  In1/1 -> Bus Creator3/1  "x_ref"
  In4/1 -> Bus Creator3/2  "y_ref"
  Derivative/1 -> Gain/1, Derivative1/1
  Derivative1/1 -> Gain1/1
  In7/1 -> conversao ref. angulos/3(psi)  "psi"
  In8/1 -> conversao ref. angulos/4(phi)  "phi"
  Gain/1 -> MATLAB Function/8(yd_dot)
  Gain1/1 -> MATLAB Function/9(yd_dotdot)
  In9/1 -> MATLAB Function/2(T)  "T"
  Constant3/1 -> MATLAB Function/10(limit)
  MATLAB Function/2(uy) -> conversao ref. angulos/2(uy)

== system SITL/Sistema de Controle do Quadrirotor/Controle/Controlador PD/Controle de Rotação/Controle de Pitch ==
  theta_ref : Inport
  theta : Inport  Port=2
  Q : Inport  Port=3
  Gain : Gain  Gain=Pitch_P
  Gain1 : Gain  Gain=-Pitch_D
  Scope3 : Scope
      settings: YMin=37.75  YMax=40  SaveName=ScopeData3
  Sum : Sum  Inputs=|+-
  Sum1 : Sum  Inputs=|++
  U_pitch : Outport
  wires:
  Sum/1 -> Gain/1
  theta_ref/1 -> Sum/1  "theta_ref"
  Sum1/1 -> Scope3/1, U_pitch/1
  Gain/1 -> Sum1/1
  theta/1 -> Sum/2
  Gain1/1 -> Sum1/2
  Q/1 -> Gain1/1

== system SITL/Sistema de Controle do Quadrirotor/Controle/Controlador PD/Controle de Rotação/Controle de Roll ==
  phi_ref : Inport
  phi : Inport  Port=2
  P : Inport  Port=3
  Gain : Gain  Gain=Roll_P
  Gain1 : Gain  Gain=-Roll_D
  Scope3 : Scope
      settings: YMin=-2500  YMax=2500  SaveName=ScopeData3
  Sum : Sum  Inputs=|+-
  Sum1 : Sum  Inputs=|++
  U_roll : Outport
  wires:
  Sum/1 -> Gain/1
  P/1 -> Gain1/1
  Gain/1 -> Sum1/1
  Gain1/1 -> Sum1/2
  Sum1/1 -> Scope3/1, U_roll/1
  phi_ref/1 -> Sum/1  "phi_ref"
  phi/1 -> Sum/2

== system SITL/Sistema de Controle do Quadrirotor/Controle/Controlador PD/Controle de Rotação/Controle de Yaw ==
  psi_ref : Inport
  psi : Inport  Port=2
  R : Inport  Port=3
  Gain : Gain  Gain=Yaw_P
  Gain1 : Gain  Gain=-Yaw_D
  Scope3 : Scope
      settings: YMin=37.75  YMax=40  SaveName=ScopeData3
  Sum : Sum  Inputs=|+-
  Sum1 : Sum  Inputs=|++
  U_yaw : Outport
  wires:
  Sum/1 -> Gain/1
  Sum1/1 -> Scope3/1, U_yaw/1
  psi/1 -> Sum/2
  psi_ref/1 -> Sum/1  "psi_ref"
  Gain/1 -> Sum1/1
  R/1 -> Gain1/1
  Gain1/1 -> Sum1/2

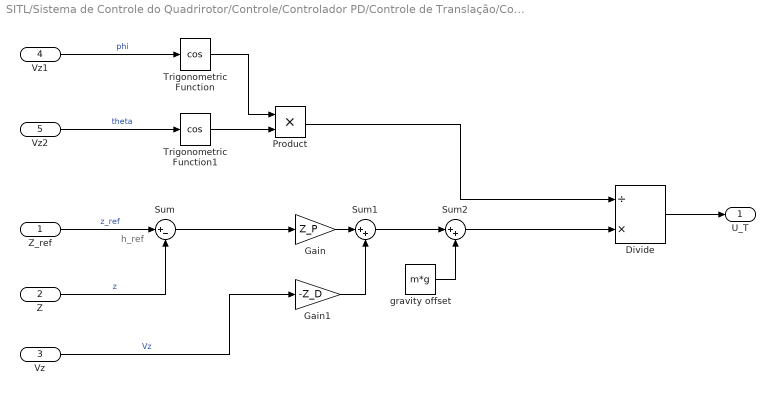
== system SITL/Sistema de Controle do Quadrirotor/Controle/Controlador PD/Controle de Translação/Controle de Altitude ==
  note: h_ref
  Z_ref : Inport
  Z : Inport  Port=2
  Vz : Inport  Port=3
  Vz1 : Inport  Port=4
  Vz2 : Inport  Port=5
  Divide : Product  Inputs=/*
  Gain : Gain  Gain=Z_P
  Gain1 : Gain  Gain=-Z_D
  Product : Product
  Sum : Sum  Inputs=|+-
  Sum1 : Sum  Inputs=|++
  Sum2 : Sum  Inputs=|++
  Trigonometric Function : Trigonometry  Operator=cos
  Trigonometric Function1 : Trigonometry  Operator=cos
  gravity offset : Constant  Value=m*g
  U_T : Outport
  wires:
  Sum/1 -> Gain/1
  Sum2/1 -> Divide/2
  Vz/1 -> Gain1/1  "Vz"
  gravity offset/1 -> Sum2/2
  Z_ref/1 -> Sum/1  "z_ref"
  Z/1 -> Sum/2  "z"
  Gain/1 -> Sum1/1
  Gain1/1 -> Sum1/2
  Sum1/1 -> Sum2/1
  Trigonometric Function1/1 -> Product/2
  Trigonometric Function/1 -> Product/1
  Product/1 -> Divide/1
  Divide/1 -> U_T/1
  Vz1/1 -> Trigonometric Function/1  "phi"
  Vz2/1 -> Trigonometric Function1/1  "theta"

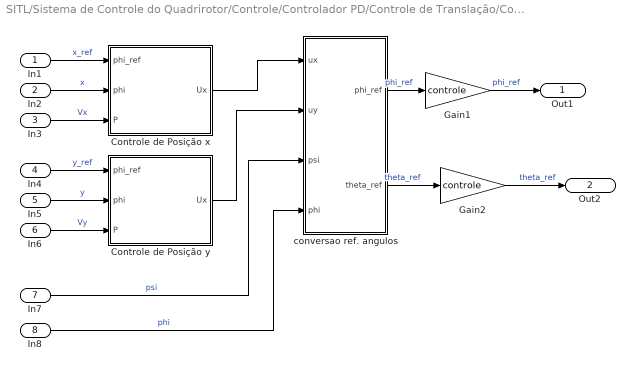
== system SITL/Sistema de Controle do Quadrirotor/Controle/Controlador PD/Controle de Translação/Controle de Posição ==
  In1 : Inport
  In2 : Inport  Port=2
  In3 : Inport  Port=3
  In4 : Inport  Port=4
  In5 : Inport  Port=5
  In6 : Inport  Port=6
  In7 : Inport  Port=7
  In8 : Inport  Port=8
  Controle de Posição x : Subsystem
  Controle de Posição y : Subsystem
  Gain1 : Gain  Gain=controle
  Gain2 : Gain  Gain=controle
  conversao ref. angulos : MATLAB Function  TreatAsAtomicUnit=on
  Out1 : Outport
  Out2 : Outport  Port=2
  wires:
  In1/1 -> Controle de Posição x/1(phi_ref)  "x_ref"
  In5/1 -> Controle de Posição y/2(phi)  "y"
  In2/1 -> Controle de Posição x/2(phi)  "x"
  In4/1 -> Controle de Posição y/1(phi_ref)  "y_ref"
  In6/1 -> Controle de Posição y/3(P)  "Vy"
  In3/1 -> Controle de Posição x/3(P)  "Vx"
  conversao ref. angulos/1(phi_ref) -> Gain1/1  "phi_ref"
  conversao ref. angulos/2(theta_ref) -> Gain2/1  "theta_ref"
  Controle de Posição x/1(Ux) -> conversao ref. angulos/1(ux)
  Controle de Posição y/1(Ux) -> conversao ref. angulos/2(uy)
  In7/1 -> conversao ref. angulos/3(psi)  "psi"
  In8/1 -> conversao ref. angulos/4(phi)  "phi"
  Gain1/1 -> Out1/1  "phi_ref"
  Gain2/1 -> Out2/1  "theta_ref"

== system SITL/Sistema de Controle do Quadrirotor/Controle/Controlador PD/Controle de Translação/Controle de Posição/Controle de Posição x ==
  phi_ref : Inport
  phi : Inport  Port=2
  P : Inport  Port=3
  Gain : Gain  Gain=pos_P
  Gain1 : Gain  Gain=-pos_D
  Gain2 : Gain  Gain=controle
  Sum : Sum  Inputs=|+-
  Sum1 : Sum  Inputs=|++
  Ux : Outport
  wires:
  Sum/1 -> Gain/1
  P/1 -> Gain1/1  "Vx"
  Gain/1 -> Sum1/1
  Gain1/1 -> Sum1/2
  Sum1/1 -> Gain2/1  "Ux"
  phi_ref/1 -> Sum/1  "x_ref"
  phi/1 -> Sum/2  "x"
  Gain2/1 -> Ux/1

== system SITL/Sistema de Controle do Quadrirotor/Controle/Controlador PD/Controle de Translação/Controle de Posição/Controle de Posição y ==
  phi_ref : Inport
  phi : Inport  Port=2
  P : Inport  Port=3
  Gain : Gain  Gain=pos_P
  Gain1 : Gain  Gain=-pos_D
  Gain2 : Gain  Gain=controle
  Sum : Sum  Inputs=|+-
  Sum1 : Sum  Inputs=|++
  Ux : Outport
  wires:
  Sum/1 -> Gain/1
  P/1 -> Gain1/1  "Vy"
  Gain/1 -> Sum1/1
  Gain1/1 -> Sum1/2
  Sum1/1 -> Gain2/1  "Uy"
  phi_ref/1 -> Sum/1  "y_ref"
  phi/1 -> Sum/2  "y"
  Gain2/1 -> Ux/1

== matlab function SITL/X-Plane Quadrirotor UDP Receiver/Embedded MATLAB Function1 ==
  data: data_in input; X output; Y output; Z output; Vx output; Vy output; Vz output; q output; p output; r output; pitch output; roll output; heading_true output
function [X, Y, Z, Vx, Vy, Vz, q, p, r, pitch, roll, heading_true]   = fcn(data_in)

% data_in(a,b)
% a = number of the byte of the packet (the packet sent from X-Plane goes from 2 to 9, that are the intances)
% b = number of the the label selected on X-Plane (in this case it was selected 3 labels, so it goes from 1 to 3)

q = data_in(2,1);
p = data_in(3,1);
r = data_in(4,1);

pitch = data_in(2,2);
roll = data_in(3,2);
heading_true = data_in(4,2);

X = data_in(2,3);
Y = data_in(3,3);
Z = data_in(4,3);

Vx = data_in(5,3);
Vy = data_in(6,3);
Vz = data_in(7,3);

== matlab function SITL/Sistema de Controle do Quadrirotor/Conversão dos comandos/MATLAB Function ==
  data: u_T input; w1d output; u_L input; u_M input; u_N input; w2d output; w3d output; w4d output; d input; ct input; cq input
function [w1d,w2d,w3d,w4d] = commands_conv(u_T,u_L,u_M,u_N,d,ct,cq)


u_z = u_T/(4*ct);
u_phi = u_L/(2*d*ct);
u_theta = u_M/(2*d*ct);
u_psi = u_N/(4*cq);

w1d_sq=u_z+u_theta+u_psi;
w2d_sq=u_z-u_phi-u_psi;
w3d_sq=u_z-u_theta+u_psi;
w4d_sq=u_z+u_phi-u_psi;


if w1d_sq<0
    w1d_sq=0;
end
if w2d_sq<0
    w2d_sq=0;
end
if w3d_sq<0
    w3d_sq=0;
end
if w4d_sq<0
    w4d_sq=0;
end



w1d = sqrt(w1d_sq);
w2d = sqrt(w2d_sq);
w3d = sqrt(w3d_sq);
w4d = sqrt(w4d_sq);

== matlab function SITL/Sistema de Controle do Quadrirotor/Motores/Motor 1/MATLAB Function ==
  data: wd input; w input; ke input; cq input; kt input; R input; Ja input; wder output
function wder = motor(wd,w,ke,cq,kt,R,Ja)

wss = wd;

V = ke*wss + (cq*R/kt)*wss^2;

wder = -(kt*ke*w)/(R*Ja) - (cq*w^2/Ja) + (kt*V)/(Ja*R);

== matlab function SITL/X-Plane Quadrirotor UDP Sender/MATLAB Function ==
  data: throttle1 input; header output single size=1; throttle_cmd output size=[1 18]; throttle2 input; throttle3 input; throttle4 input
function [header, throttle_cmd]  = fcn(throttle1, throttle2, throttle3, throttle4)

%The header have 4 bytes plus one byte with 0

header = typecast(uint8([uint8(68) uint8(65) uint8(84) uint8(65)]), 'single');

%To send no comand for the instances we dont need to use, it is used -999

No_Comand = single(-999);

%The first group of four bytes in a selected field presents a label to identify the set of data(in this case throttle). 
%The second group has the first instance of the data set ;
%The third group has the second instance, etc. (Throttle1, 2, 3 and 4) 

Throttle_header = typecast(uint8([uint8(25) uint8(0) uint8(0) uint8(0)]), 'single');
throttle_cmd = [Throttle_header throttle1 throttle2 throttle3 throttle4 No_Comand No_Comand No_Comand No_Comand Throttle_header No_Comand No_Comand No_Comand No_Comand No_Comand No_Comand No_Comand No_Comand];

== matlab function SITL/Sistema de Controle do Quadrirotor/Motores/Motor 2/MATLAB Function ==
  data: wd input; w input; ke input; cq input; kt input; R input; Ja input; wder output
function wder = motor(wd,w,ke,cq,kt,R,Ja)

wss = wd;

V = ke*wss + (cq*R/kt)*wss^2;

wder = -(kt*ke*w)/(R*Ja) - (cq*w^2/Ja) + (kt*V)/(Ja*R);

== matlab function SITL/Sistema de Controle do Quadrirotor/Motores/Motor 3/MATLAB Function ==
  data: wd input; w input; ke input; cq input; kt input; R input; Ja input; wder output
function wder = motor(wd,w,ke,cq,kt,R,Ja)

wss = wd;

V = ke*wss + (cq*R/kt)*wss^2;

wder = -(kt*ke*w)/(R*Ja) - (cq*w^2/Ja) + (kt*V)/(Ja*R);

== matlab function SITL/Sistema de Controle do Quadrirotor/Controle/Controlador PD/Controle de Translação/Controle de Posição/conversao ref. angulos ==
  data: ux input; uy input; psi input; phi input; phi_ref output; theta_ref output
function [phi_ref,theta_ref] = conv_ang_ref(ux,uy,psi,phi)

arg_phi = ux*sin(psi)-uy*cos(psi);

if arg_phi>1
    arg_phi=1;
elseif arg_phi<-1
    arg_phi=-1;
end

arg_theta = (ux*cos(psi)+uy*sin(psi))/(cos(phi));

if arg_theta>1
    arg_theta=1;
elseif arg_theta<-1
    arg_theta=-1;
end


phi_ref = asin(arg_phi);

theta_ref = asin(arg_theta);

== matlab function SITL/Sistema de Controle do Quadrirotor/Controle/Controlador sliding mode/MATLAB Function ==
  data: u_T output; u_L output; g input; J input; m input; Phi input; Theta input; Psi input; y input; y_dot input; yd input; yd_dot input; yd_dotdot input; lambda input; k input; u_M output; u_N output; limit input; s output
function [u_T,u_L,u_M,u_N,s] = sliding_mode(g,J,m,Phi,Theta,Psi,y,y_dot,yd,yd_dot,yd_dotdot,lambda,k, limit)

Jxx=J(1);
Jyy=J(2);
Jzz=J(3);

lambdas = [lambda(1),0,0,0
          0,lambda(2),0,0
          0,0,lambda(3),0
          0,0,0,lambda(4)];

Phid = y_dot(2);
Thetad = y_dot(3);
Psid = y_dot(4);
      
f=zeros(4,1);

f(1)= g;

f(2)= cos(Phi)*tan(Theta)*(((Phid - Psid*sin(Theta))*(Jxx - Jyy)*(Thetad*cos(Phi) + ...
Psid*cos(Theta)*sin(Phi)))/Jzz) + sin(Phi)*tan(Theta)*(((Phid - Psid*sin(Theta))*(Jxx - Jzz)*(Thetad*sin(Phi) - Psid*cos(Phi)*cos(Theta)))/Jyy) + ...
(Psid*Thetad)/cos(Theta) + Phid*Thetad*tan(Theta) - ((Jyy - Jzz)*(Thetad*cos(Phi) + Psid*cos(Theta)*sin(Phi))*(Thetad*sin(Phi) - Psid*cos(Phi)*cos(Theta)))/Jxx;

f(3)= cos(Phi)*(((Phid - Psid*sin(Theta))*(Jxx - Jzz)*(Thetad*sin(Phi) - Psid*cos(Phi)*cos(Theta)))/Jyy) +...
    - sin(Phi)*(((Phid - Psid*sin(Theta))*(Jxx - Jyy)*(Thetad*cos(Phi) + Psid*cos(Theta)*sin(Phi)))/Jzz) - Phid*Psid*cos(Theta);

f(4) = (Phid*Thetad)/cos(Theta) + (cos(Phi)*(Jxx*(Phid - Psid*sin(Theta))*(Thetad*cos(Phi) + Psid*cos(Theta)*sin(Phi)) - Jyy*(Phid - Psid*sin(Theta))*(Thetad*cos(Phi) + Psid*cos(Theta)*sin(Phi))))/(Jzz*cos(Theta)) + ...
(sin(Phi)*(Jxx*(Phid - Psid*sin(Theta))*(Thetad*sin(Phi) - Psid*cos(Phi)*cos(Theta)) - Jzz*(Phid - Psid*sin(Theta))*(Thetad*sin(Phi) - Psid*cos(Phi)*cos(Theta))))/(Jyy*cos(Theta)) + (Psid*Thetad*sin(Theta))/cos(Theta);

s = y_dot - yd_dot + lambdas*(y - yd);


Binv=[-m/(cos(Phi)*cos(Theta)),0,0,0
       0, Jxx, 0,  -Jxx*sin(Theta)
       0, 0, (Jyy*cos(Phi)), (Jyy*cos(Theta)*sin(Phi))
       0, 0, -(Jzz*sin(Phi)), (Jzz*cos(Phi)*cos(Theta))];

k_des =  [k(1),0,0,0
          0,k(2),0,0
          0,0,k(3),0
          0,0,0,k(4)];
 
u = Binv * (-f + yd_dotdot - lambdas*(y_dot - yd_dot) - k_des * sat(s,limit));


u_T = u(1);
u_L = u(2);
u_M = u(3);
u_N = u(4);

== matlab function SITL/Sistema de Controle do Quadrirotor/Controle/Controlador sliding mode/MATLAB Function1 ==
  data: p input; phi_dot output; q input; r input; phi input; theta input; psi input; theta_dot output; psi_dot output
function [phi_dot,theta_dot,psi_dot] = pqr_to_euler_dot(p,q,r,phi,theta,psi)

phi_dot = p + tan(theta)*sin(phi)*q + tan(theta)*cos(phi)*r;

theta_dot = cos(phi)*q - sin(phi)*r;

psi_dot = q*sin(phi)/cos(theta) + r*cos(phi)/cos(theta);

== matlab function SITL/Sistema de Controle do Quadrirotor/Controle/Controlador sliding mode/Controle de Translação/conversao ref. angulos ==
  data: ux input; uy input; psi input; phi input; phi_ref output; theta_ref output
function [phi_ref,theta_ref] = conv_ang_ref(ux,uy,psi,phi)

arg_phi = ux*sin(psi)-uy*cos(psi);

if arg_phi>1
    arg_phi=1;
elseif arg_phi<-1
    arg_phi=-1;
end

arg_theta = (ux*cos(psi)+uy*sin(psi))/(cos(phi));

if arg_theta>1
    arg_theta=1;
elseif arg_theta<-1
    arg_theta=-1;
end


phi_ref = asin(arg_phi);

theta_ref = asin(arg_theta);

== matlab function SITL/Sistema de Controle do Quadrirotor/Controle/Controlador sliding mode/Controle de Translação/MATLAB Function ==
  data: m input; T input; lambda input; k input; y input; y_dot input; yd input; yd_dot input; yd_dotdot input; ux output; uy output; limit input
function [ux,uy] = posicao_sliding(m,T,lambda, k, y, y_dot, yd, yd_dot, yd_dotdot, limit)

lambdas=[lambda(1), 0
            0, lambda(2)];
        
k_des = [ k(1), 0 
             0, k(2)];
         
Binv= [-m/T, 0
        0, -m/T];
    
s = y_dot - yd_dot + lambdas*(y - yd);

u = Binv*(yd_dotdot - lambdas*(y_dot-yd_dot) - k_des*sat(s,limit));

ux=u(1);
uy=u(2);

== matlab function SITL/Sistema de Controle do Quadrirotor/Motores/Motor 4/MATLAB Function ==
  data: wd input; w input; ke input; cq input; kt input; R input; Ja input; wder output
function wder = motor(wd,w,ke,cq,kt,R,Ja)

wss = wd;

V = ke*wss + (cq*R/kt)*wss^2;

wder = -(kt*ke*w)/(R*Ja) - (cq*w^2/Ja) + (kt*V)/(Ja*R);

== matlab function SITL/Conversão Matlab2XPlane/MATLAB Function ==
  data: w1 input; t1 output; w2 input; w3 input; w4 input; t2 output; t3 output; t4 output
function [t1,t2,t3,t4] = commands_conv(w1,w2,w3,w4)

% this block is responsible for convert the angular velocity of each motor calculated on
% the control system and make it compatible with X-Plane.


w1_rpm=1.725*(60/(2*pi))*w1; % Convertion from rad/s to rpm and multiplied by a constant to make it compatible with hover velocity of X-Plane.

%t1= 0.00000000000075*w1_rpm*w1_rpm*w1_rpm;
t1= 0.0000000045*w1_rpm*w1_rpm;  % Convertion from angular velocity of the motors to thrust command. This value is sent to X-Plane.
%t1= 0.0000342*w1_rpm;


w2_rpm=1.725*(60/(2*pi))*w2;

%t2= 0.00000000000075*w2_rpm*w2_rpm*w2_rpm;
t2= 0.0000000045*w2_rpm*w2_rpm;
%t2= 0.0000342*w2_rpm;


w3_rpm=1.725*(60/(2*pi))*w3;

%t3= 0.00000000000075*w3_rpm*w3_rpm*w3_rpm;
t3= 0.0000000045*w3_rpm*w3_rpm;
%t3= 0.0000342*w3_rpm;


w4_rpm=1.725*(60/(2*pi))*w4;

%t4= 0.00000000000075*w4_rpm*w4_rpm*w4_rpm;
t4= 0.0000000045*w4_rpm*w4_rpm;
%t4= 0.0000342*w4_rpm;

== matlab function SITL/Conversão XPlane2Matlab/MATLAB Function ==
  data: X_XPlane input; X output; Y_XPlane input; Z_XPlane input; Vx_XPlane input; Y output; Z output; Vx output; Vy output; Vz output; q output; p output; r output; theta output; phi output; psi output; Vy_XPlane input; Vz_XPlane input; q_XPlane input; p_XPlane input; r_XPlane input; pitch_XPlane input; roll_XPlane input; heading_XPlane input
function [X,Y,Z,Vx,Vy,Vz,q,p,r,theta,phi,psi] = commands_conv(X_XPlane,Y_XPlane,Z_XPlane,Vx_XPlane,Vy_XPlane,Vz_XPlane,q_XPlane,p_XPlane,r_XPlane,pitch_XPlane,roll_XPlane,heading_XPlane)

%this block is responsible to make the variables of Xplane compatible with
%the variables of the control system.

X0=-35162.53;  %Initial position of the Quadcopter on X-Plane 
Y0=180.60;     %TODO: Get the values autonomously
Z0=2784.36;


X=-Z_XPlane-(-Z0); % CONVERTION FOR NED SYSTEM
Y=X_XPlane-(X0);
Z=-Y_XPlane-(-Y0);

Vx=-Vz_XPlane; % CONVERTION FOR NED SYSTEM 
Vy=Vx_XPlane;
Vz=-Vy_XPlane;

q=q_XPlane; % EQUAL
p=p_XPlane;
r=r_XPlane;

theta=pitch_XPlane*(pi/180); % CONVERTION FROM DEG TO RAD
phi=roll_XPlane*(pi/180);
psi=heading_XPlane*(pi/180);
